simulink model "frontierdemo"  (R2025b)
settings: Solver=FixedStepAuto  StartTime=0.0  StopTime=inf  FixedStep=0.05  RelTol=1e-3
libraries: robotlib x6
settings Model: Creator=sprinkle  LastModifiedBy=sanborkl
settings OptimizationCC: DefaultParameterBehavior=Inlined  EnhancedBackFolding=on  PassReuseOutputArgsAs=Individual arguments  ZeroExternalMemoryAtStartup=off  ZeroInternalMemoryAtStartup=off  MaxStackSize=64  OptimizeBlockOrder=speed  DifferentSizesBufferReuse=on  OptimizationCustomize=off  EfficientTunableParamExpr=on
settings DebuggingCC: ParameterTunabilityLossMsg=error
settings HardwareCC: ProdBitPerPointer=32.0  ProdBitPerSizeT=32.0  ProdBitPerPtrDiffT=32.0  ProdLargestAtomicFloat=None  ProdIntDivRoundTo=Undefined  ProdEndianess=Unspecified  ProdWordSize=32.0  ProdHWDeviceType=Generic->Unspecified (assume 32-bit Generic)
settings SFSimCC: MATLABDynamicMemAlloc=off
settings RTWCC: SystemTargetFile=ert.tlc  HardwareBoard=Robot Operating System (ROS)  TLCOptions="-aInlineSetEventsForThisBaseRateFcn=TLC_FALSE -aSuppressMultiTaskScheduler=TLC_FALSE  -aRateBasedStepFcn=0"  GenCodeOnly=on  TemplateMakefile=ert_default_tmf  Toolchain=Catkin  TargetLang=C++  Description=Embedded Coder
settings CodeAppCC: ForceParamTrailComments=on  IgnoreCustomStorageClasses=off  OperatorAnnotations=on  SimulinkDataObjDesc=on  SFDataObjDesc=on  InsertBlockDesc=on

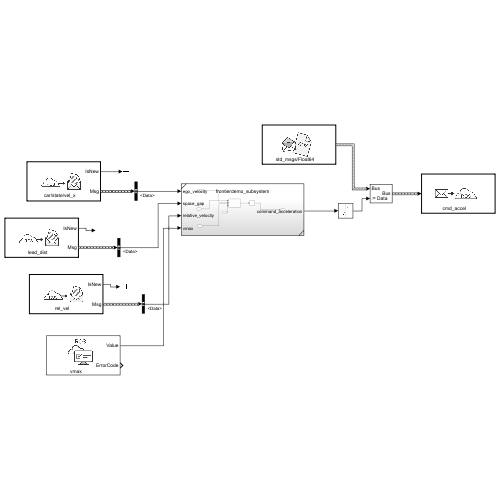
[thumbnail: Simulink's stored preview of the top-level diagram]
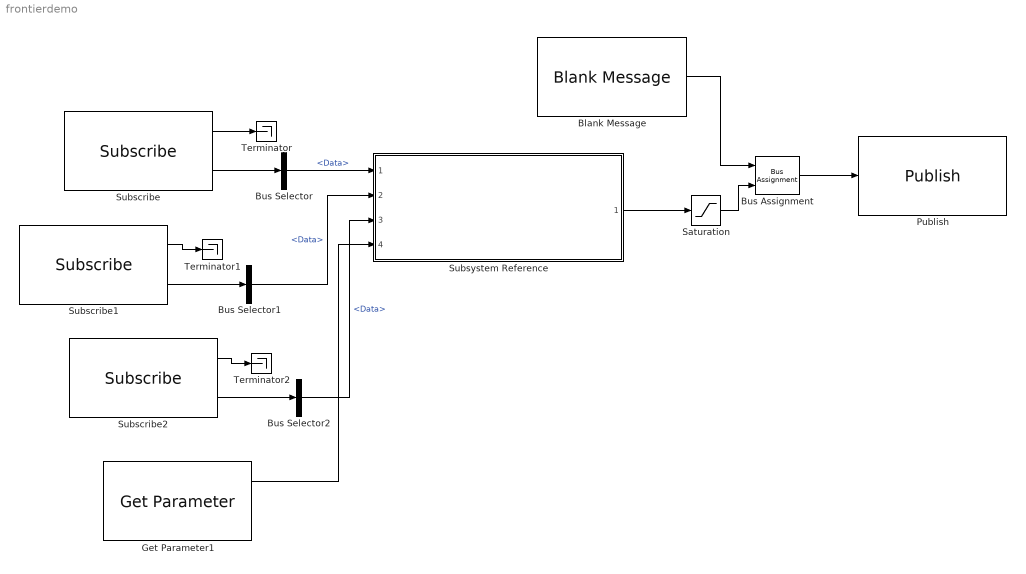
== system frontierdemo ==
  Blank Message : robotlib/Blank Message  messageClass=Message  entityType=std_msgs/Float64  messageType=std_msgs/Float64  SampleTime=inf  legacyBusStruct=off
  Bus Assignment : BusAssignment  AssignedSignals=Data
  Bus Selector : BusSelector  OutputSignals=Data
  Bus Selector1 : BusSelector  OutputSignals=Data
  Bus Selector2 : BusSelector  OutputSignals=Data
  Get Parameter1 : robotlib/Get Parameter  ParameterSource=Specify your own  ParameterName=vmax  ParameterType=double  ParameterMaxArrayLength=16  ParameterInitialValue=35  SampleTime=-1  ShowErrorCodeOutput=on  ModelName=frontierdemo  BlockId=ParamGet_frontierdemo_19
  Publish : robotlib/Publish  topicSource=Specify your own  topic=cmd_accel  messageType=std_msgs/Float64  legacyBusStruct=off  messageQueueLength=1
  Saturation : Saturate  UpperLimit=1.5  LowerLimit=-3.0
  Subscribe : robotlib/Subscribe  topicSource=Specify your own  topic=car/state/vel_x  messageType=std_msgs/Float64  SampleTime=-1  legacyBusStruct=off  messageQueueLength=1
  Subscribe1 : robotlib/Subscribe  topicSource=Specify your own  topic=lead_dist  messageType=std_msgs/Float64  SampleTime=-1  legacyBusStruct=off  messageQueueLength=1
  Subscribe2 : robotlib/Subscribe  topicSource=Specify your own  topic=rel_vel  messageType=std_msgs/Float64  SampleTime=-1  legacyBusStruct=off  messageQueueLength=1
  Subsystem Reference : Subsystem  ReferencedSubsystem=frontierdemo_subsystem
  Terminator : Terminator
  Terminator1 : Terminator
  Terminator2 : Terminator
  wires:
  Subscribe/2 -> Bus Selector/1
  Subscribe/1 -> Terminator/1
  Subscribe1/2 -> Bus Selector1/1
  Subscribe1/1 -> Terminator1/1
  Blank Message/1 -> Bus Assignment/1
  Bus Assignment/1 -> Publish/1
  Bus Selector1/1 -> Subsystem Reference/2  "<Data>"
  Bus Selector/1 -> Subsystem Reference/1  "<Data>"
  Get Parameter1/1 -> Subsystem Reference/4
  Saturation/1 -> Bus Assignment/2
  Subsystem Reference/1 -> Saturation/1
  Subscribe2/2 -> Bus Selector2/1
  Bus Selector2/1 -> Subsystem Reference/3  "<Data>"
  Subscribe2/1 -> Terminator2/1
